simulink model "schemablocpunctb"  (R2021b)
settings: Solver=VariableStepAuto  StartTime=0.0  StopTime=10.0  RelTol=1e-3
model workspace (MAT data in the model file):
  a = Simulink.Parameter
  a.DataType = 'auto'
  a.Complexity = 'real'
  a.Dimensions = [0 0]

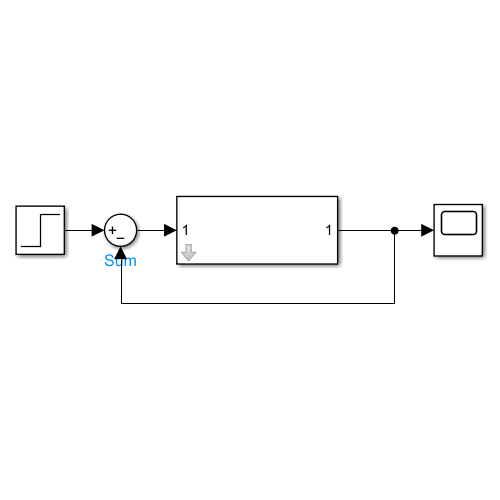
[thumbnail: Simulink's stored preview of the top-level diagram]
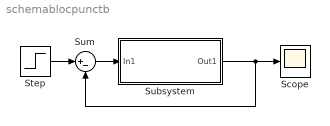
== system schemablocpunctb ==
  Scope : Scope
  Step : Step  SampleTime=0
  Subsystem : Subsystem  mask{a=6}
      mask Callback a:
      | if str2num(get_param(gcb, 'a'))<6
      |     error('amplitudinea este diferita de constrangeri')
      | end
      | if str2num(get_param(gcb, 'a'))>8
      |     error('amplitudinea este diferita de constrangeri')
      | end
  Sum : Sum  Inputs=|+-
  wires:
  Subsystem/1(Out1) -> Sum/2, Scope/1
  Step/1 -> Sum/1
  Sum/1 -> Subsystem/1(In1)

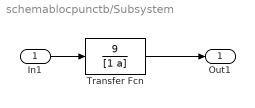
== system schemablocpunctb/Subsystem ==
  In1 : Inport
  Transfer Fcn : TransferFcn  Numerator=[9]  Denominator=[1 a]
  Out1 : Outport
  wires:
  In1/1 -> Transfer Fcn/1
  Transfer Fcn/1 -> Out1/1
